simulink model "XYctrl_obs_avoid"  (Simulink 8.1)
settings: Solver=ode45  StartTime=0.0  StopTime=10.0  RelTol=1e-3
values from neighbouring files (symbols this model uses):
  XYctrl =     [XYctrl_ObstAvoidance.mat]
settings Model: Creator=Atum  LastModifiedBy=Kostas
settings DebuggingCC: FcnCallInpInsideContextMsg=EnableAllAsWarning
settings GRTTargetCC: CombineOutputUpdateFcns=on  GRTInterface=off

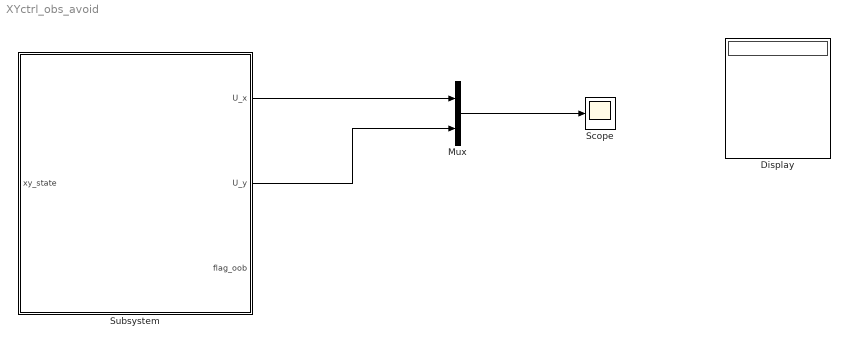
== system XYctrl_obs_avoid ==
  Display : Display
  Mux : Mux  Inputs=2
  Scope : Scope
      settings: SaveName=Uxy
  Subsystem : Subsystem
  wires:
  Subsystem/1(U_x) -> Mux/1
  Subsystem/2(U_y) -> Mux/2
  Mux/1 -> Scope/1
  ? -> Subsystem/1(xy_state)

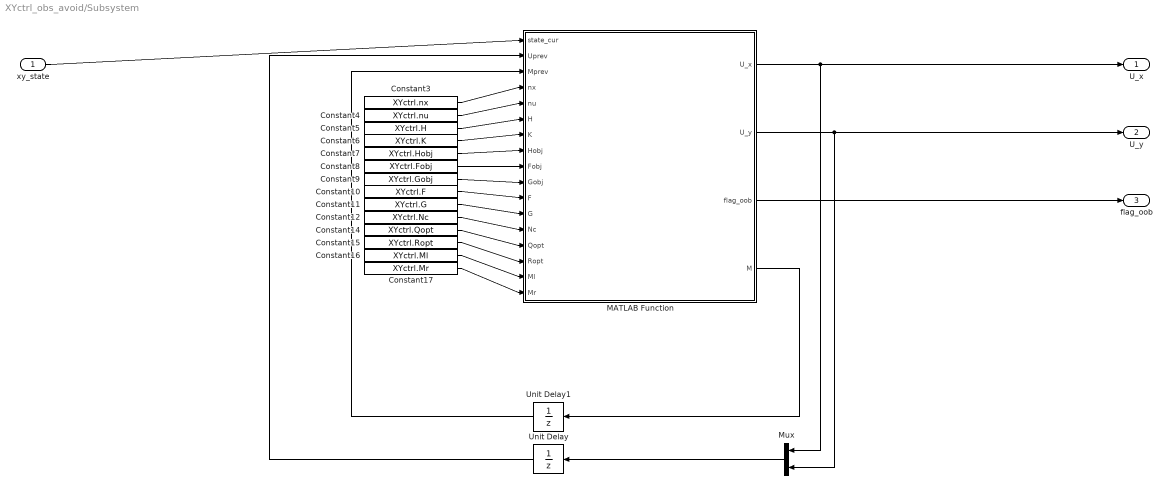
== system XYctrl_obs_avoid/Subsystem ==
  xy_state : Inport
  Constant10 : Constant  Value=XYctrl.F  VectorParams1D=off
  Constant11 : Constant  Value=XYctrl.G  VectorParams1D=off
  Constant12 : Constant  Value=XYctrl.Nc  VectorParams1D=off
  Constant14 : Constant  Value=XYctrl.Qopt  VectorParams1D=off
  Constant15 : Constant  Value=XYctrl.Ropt  VectorParams1D=off
  Constant16 : Constant  Value=XYctrl.Ml  VectorParams1D=off
  Constant17 : Constant  Value=XYctrl.Mr  VectorParams1D=off
  Constant3 : Constant  Value=XYctrl.nx  VectorParams1D=off
  Constant4 : Constant  Value=XYctrl.nu  VectorParams1D=off
  Constant5 : Constant  Value=XYctrl.H  VectorParams1D=off
  Constant6 : Constant  Value=XYctrl.K  VectorParams1D=off
  Constant7 : Constant  Value=XYctrl.Hobj  VectorParams1D=off
  Constant8 : Constant  Value=XYctrl.Fobj  VectorParams1D=off
  Constant9 : Constant  Value=XYctrl.Gobj  VectorParams1D=off
  MATLAB Function : MATLAB Function  TreatAsAtomicUnit=on
  Mux : Mux  Inputs=2
  Unit Delay : UnitDelay  InitialCondition=[0 0]  SampleTime=-1
  Unit Delay1 : UnitDelay  InitialCondition=1  SampleTime=-1
  U_x : Outport
  U_y : Outport  Port=2
  flag_oob : Outport  Port=3
  wires:
  Constant3/1 -> MATLAB Function/4(nx)
  MATLAB Function/4(M) -> Unit Delay1/1
  Constant4/1 -> MATLAB Function/5(nu)
  Constant5/1 -> MATLAB Function/6(H)
  Constant6/1 -> MATLAB Function/7(K)
  Constant7/1 -> MATLAB Function/8(Hobj)
  Constant8/1 -> MATLAB Function/9(Fobj)
  Constant9/1 -> MATLAB Function/10(Gobj)
  Constant10/1 -> MATLAB Function/11(F)
  Constant11/1 -> MATLAB Function/12(G)
  Constant12/1 -> MATLAB Function/13(Nc)
  Constant14/1 -> MATLAB Function/14(Qopt)
  Constant15/1 -> MATLAB Function/15(Ropt)
  Constant16/1 -> MATLAB Function/16(Ml)
  Constant17/1 -> MATLAB Function/17(Mr)
  xy_state/1 -> MATLAB Function/1(state_cur)
  Mux/1 -> Unit Delay/1
  MATLAB Function/1(U_x) -> Mux/1, U_x/1
  MATLAB Function/2(U_y) -> Mux/2, U_y/1
  Unit Delay/1 -> MATLAB Function/2(Uprev)
  Unit Delay1/1 -> MATLAB Function/3(Mprev)
  MATLAB Function/3(flag_oob) -> flag_oob/1

== matlab function Subsystem/MATLAB Function ==
  data: state_cur input double; U_x output double; Uprev input double; Mprev input double; nx input double; nu input double; H input double; K input double; Hobj input double; Fobj input double; Gobj input double; F input double; G input double; Nc input double; Qopt input double; Ropt input double; Ml input double; Mr input double; U_y output double; flag_oob output double; M output double
function [U_x,U_y,flag_oob,M] = fcn(state_cur,Uprev,Mprev,nx,nu,H,K,Hobj,Fobj,Gobj,F,G,Nc,Qopt,Ropt,Ml,Mr)
%#codegen

[U,flag_oob,M] = OptimalMPCInputExportC_vP(state_cur,Uprev,Mprev,nx,nu,H,K,Hobj,Fobj,Gobj,F,G,Nc,Qopt,Ropt,Ml,Mr)

U_x = U(1);
U_y = U(2);

end
